simulink model "UberSpurs"  (R2015b)
settings: Solver=VariableStepAuto  StartTime=0.0  StopTime=10000  RelTol=1e-3
(part 4 of 4)

== stateflow chart UberSpurs/spur1WorkCell/route2Channel9/RoutingControlBehavior ==
  (default) -> (junction 7) : % toChanel
  (junction 7) -> (junction 8) [order 1] : [entityChannel == channel && serverAvailable ==0]
  (junction 7) -> (junction 9) [order 2] : {route = 2;}
  (junction 8) -> (junction 10) : {route = 1 ;}
  (junction 10) -> (junction 9)
  (junction 9) -> (junction 11)
  data: entityChannel input; channel input; route output; serverAvailable input

== stateflow chart UberSpurs/spur1WorkCell/route2recirculate/Chart ==
  (default) -> (junction 7) : % recirculate
  (junction 7) -> (junction 9) [order 1] : [FillTime>0]
  (junction 9) -> (junction 23) [order 1] : [verifyQueue<6]
  (junction 9) -> (junction 20) [order 2] : {route = 1;}
  (junction 7) -> (junction 8) [order 2] : {route = 1;}
  (junction 23) -> (junction 25) : {route = 2;}
  (junction 20) -> (junction 8)
  (junction 25) -> (junction 20)
  (junction 8) -> (junction 11)
  data: FillTime input; route output; verifyQueue input

== stateflow chart UberSpurs/AdmissionControlBehavior ==
  (default) -> (junction 7) : % wipLimit
  (junction 7) -> (junction 8) [order 1] : [WIP <= 120]
  (junction 7) -> (junction 9) [order 2] : {admission = 0;}
  (junction 8) -> (junction 10) : {admission = 1;}
  (junction 10) -> (junction 9)
  (junction 9) -> (junction 11)
  data: WIP input; admission output

== stateflow chart UberSpurs/spur1WorkCell/route2Channel10/RoutingControlBehavior ==
  (default) -> (junction 7) : % toChanel
  (junction 7) -> (junction 8) [order 1] : [entityChannel == channel && serverAvailable ==0]
  (junction 7) -> (junction 9) [order 2] : {route = 2;}
  (junction 8) -> (junction 10) : {route = 1 ;}
  (junction 10) -> (junction 9)
  (junction 9) -> (junction 11)
  data: entityChannel input; channel input; route output; serverAvailable input

== stateflow chart UberSpurs/spur1WorkCell/route2Channel11/RoutingControlBehavior ==
  (default) -> (junction 7) : % toChanel
  (junction 7) -> (junction 8) [order 1] : [entityChannel == channel && serverAvailable ==0]
  (junction 7) -> (junction 9) [order 2] : {route = 2;}
  (junction 8) -> (junction 10) : {route = 1 ;}
  (junction 10) -> (junction 9)
  (junction 9) -> (junction 11)
  data: entityChannel input; channel input; route output; serverAvailable input

== stateflow chart UberSpurs/spur1WorkCell/route2Channel12/RoutingControlBehavior ==
  (default) -> (junction 7) : % toChanel
  (junction 7) -> (junction 8) [order 1] : [entityChannel == channel && serverAvailable ==0]
  (junction 7) -> (junction 9) [order 2] : {route = 2;}
  (junction 8) -> (junction 10) : {route = 1 ;}
  (junction 10) -> (junction 9)
  (junction 9) -> (junction 11)
  data: entityChannel input; channel input; route output; serverAvailable input

== stateflow chart UberSpurs/spur1WorkCell/route2Channel13/RoutingControlBehavior ==
  (default) -> (junction 7) : % toChanel
  (junction 7) -> (junction 8) [order 1] : [entityChannel == channel && serverAvailable ==0]
  (junction 7) -> (junction 9) [order 2] : {route = 2;}
  (junction 8) -> (junction 10) : {route = 1 ;}
  (junction 10) -> (junction 9)
  (junction 9) -> (junction 11)
  data: entityChannel input; channel input; route output; serverAvailable input

== stateflow chart UberSpurs/spur1WorkCell/route2Channel14/RoutingControlBehavior ==
  (default) -> (junction 7) : % toChanel
  (junction 7) -> (junction 8) [order 1] : [entityChannel == channel && serverAvailable ==0]
  (junction 7) -> (junction 9) [order 2] : {route = 2;}
  (junction 8) -> (junction 10) : {route = 1 ;}
  (junction 10) -> (junction 9)
  (junction 9) -> (junction 11)
  data: entityChannel input; channel input; route output; serverAvailable input

== stateflow chart UberSpurs/spur1WorkCell/route2Channel15/RoutingControlBehavior ==
  (default) -> (junction 7) : % toChanel
  (junction 7) -> (junction 8) [order 1] : [entityChannel == channel && serverAvailable ==0]
  (junction 7) -> (junction 9) [order 2] : {route = 2;}
  (junction 8) -> (junction 10) : {route = 1 ;}
  (junction 10) -> (junction 9)
  (junction 9) -> (junction 11)
  data: entityChannel input; channel input; route output; serverAvailable input

== stateflow chart UberSpurs/spur1WorkCell/route2Channel16/RoutingControlBehavior ==
  (default) -> (junction 7) : % toChanel
  (junction 7) -> (junction 8) [order 1] : [entityChannel == channel && serverAvailable ==0]
  (junction 7) -> (junction 9) [order 2] : {route = 2;}
  (junction 8) -> (junction 10) : {route = 1 ;}
  (junction 10) -> (junction 9)
  (junction 9) -> (junction 11)
  data: entityChannel input; channel input; route output; serverAvailable input

== stateflow chart UberSpurs/spur1WorkCell/route2Channel17/RoutingControlBehavior ==
  (default) -> (junction 7) : % toChanel
  (junction 7) -> (junction 8) [order 1] : [entityChannel == channel && serverAvailable ==0]
  (junction 7) -> (junction 9) [order 2] : {route = 2;}
  (junction 8) -> (junction 10) : {route = 1 ;}
  (junction 10) -> (junction 9)
  (junction 9) -> (junction 11)
  data: entityChannel input; channel input; route output; serverAvailable input

== stateflow chart UberSpurs/spur1WorkCell/route2Channel18/RoutingControlBehavior ==
  (default) -> (junction 7) : % toChanel
  (junction 7) -> (junction 8) [order 1] : [entityChannel == channel && serverAvailable ==0]
  (junction 7) -> (junction 9) [order 2] : {route = 2;}
  (junction 8) -> (junction 10) : {route = 1 ;}
  (junction 10) -> (junction 9)
  (junction 9) -> (junction 11)
  data: entityChannel input; channel input; route output; serverAvailable input

== stateflow chart UberSpurs/route2Spur2/routingControl ==
  (default) -> (junction 9) : % route2Spur
  (junction 9) -> (junction 10) [order 1] : [entitySpur == 2]
  (junction 9) -> (junction 11) [order 2] : {route = 1;}
  (junction 10) -> (junction 12) : {route = 2;}
  (junction 12) -> (junction 11)
  (junction 11) -> (junction 13)
  data: entitySpur input; route output

== stateflow chart UberSpurs/spur2WorkCell/route2Channel1/RoutingControlBehavior ==
  (default) -> (junction 7) : % toChanel
  (junction 7) -> (junction 8) [order 1] : [entityChannel == channel && serverAvailable ==0]
  (junction 7) -> (junction 9) [order 2] : {route = 2;}
  (junction 8) -> (junction 10) : {route = 1 ;}
  (junction 10) -> (junction 9)
  (junction 9) -> (junction 11)
  data: entityChannel input; channel input; route output; serverAvailable input

== stateflow chart UberSpurs/spur2WorkCell/route2Channel10/RoutingControlBehavior ==
  (default) -> (junction 7) : % toChanel
  (junction 7) -> (junction 8) [order 1] : [entityChannel == channel && serverAvailable ==0]
  (junction 7) -> (junction 9) [order 2] : {route = 2;}
  (junction 8) -> (junction 10) : {route = 1 ;}
  (junction 10) -> (junction 9)
  (junction 9) -> (junction 11)
  data: entityChannel input; channel input; route output; serverAvailable input

== stateflow chart UberSpurs/spur2WorkCell/route2Channel11/RoutingControlBehavior ==
  (default) -> (junction 7) : % toChanel
  (junction 7) -> (junction 8) [order 1] : [entityChannel == channel && serverAvailable ==0]
  (junction 7) -> (junction 9) [order 2] : {route = 2;}
  (junction 8) -> (junction 10) : {route = 1 ;}
  (junction 10) -> (junction 9)
  (junction 9) -> (junction 11)
  data: entityChannel input; channel input; route output; serverAvailable input

== stateflow chart UberSpurs/spur2WorkCell/route2Channel12/RoutingControlBehavior ==
  (default) -> (junction 7) : % toChanel
  (junction 7) -> (junction 8) [order 1] : [entityChannel == channel && serverAvailable ==0]
  (junction 7) -> (junction 9) [order 2] : {route = 2;}
  (junction 8) -> (junction 10) : {route = 1 ;}
  (junction 10) -> (junction 9)
  (junction 9) -> (junction 11)
  data: entityChannel input; channel input; route output; serverAvailable input

== stateflow chart UberSpurs/spur2WorkCell/route2Channel13/RoutingControlBehavior ==
  (default) -> (junction 7) : % toChanel
  (junction 7) -> (junction 8) [order 1] : [entityChannel == channel && serverAvailable ==0]
  (junction 7) -> (junction 9) [order 2] : {route = 2;}
  (junction 8) -> (junction 10) : {route = 1 ;}
  (junction 10) -> (junction 9)
  (junction 9) -> (junction 11)
  data: entityChannel input; channel input; route output; serverAvailable input

== stateflow chart UberSpurs/spur2WorkCell/route2Channel14/RoutingControlBehavior ==
  (default) -> (junction 7) : % toChanel
  (junction 7) -> (junction 8) [order 1] : [entityChannel == channel && serverAvailable ==0]
  (junction 7) -> (junction 9) [order 2] : {route = 2;}
  (junction 8) -> (junction 10) : {route = 1 ;}
  (junction 10) -> (junction 9)
  (junction 9) -> (junction 11)
  data: entityChannel input; channel input; route output; serverAvailable input

== stateflow chart UberSpurs/spur2WorkCell/route2Channel15/RoutingControlBehavior ==
  (default) -> (junction 7) : % toChanel
  (junction 7) -> (junction 8) [order 1] : [entityChannel == channel && serverAvailable ==0]
  (junction 7) -> (junction 9) [order 2] : {route = 2;}
  (junction 8) -> (junction 10) : {route = 1 ;}
  (junction 10) -> (junction 9)
  (junction 9) -> (junction 11)
  data: entityChannel input; channel input; route output; serverAvailable input

== stateflow chart UberSpurs/spur2WorkCell/route2Channel16/RoutingControlBehavior ==
  (default) -> (junction 7) : % toChanel
  (junction 7) -> (junction 8) [order 1] : [entityChannel == channel && serverAvailable ==0]
  (junction 7) -> (junction 9) [order 2] : {route = 2;}
  (junction 8) -> (junction 10) : {route = 1 ;}
  (junction 10) -> (junction 9)
  (junction 9) -> (junction 11)
  data: entityChannel input; channel input; route output; serverAvailable input

== stateflow chart UberSpurs/spur2WorkCell/route2Channel17/RoutingControlBehavior ==
  (default) -> (junction 7) : % toChanel
  (junction 7) -> (junction 8) [order 1] : [entityChannel == channel && serverAvailable ==0]
  (junction 7) -> (junction 9) [order 2] : {route = 2;}
  (junction 8) -> (junction 10) : {route = 1 ;}
  (junction 10) -> (junction 9)
  (junction 9) -> (junction 11)
  data: entityChannel input; channel input; route output; serverAvailable input

== stateflow chart UberSpurs/spur2WorkCell/route2Channel18/RoutingControlBehavior ==
  (default) -> (junction 7) : % toChanel
  (junction 7) -> (junction 8) [order 1] : [entityChannel == channel && serverAvailable ==0]
  (junction 7) -> (junction 9) [order 2] : {route = 2;}
  (junction 8) -> (junction 10) : {route = 1 ;}
  (junction 10) -> (junction 9)
  (junction 9) -> (junction 11)
  data: entityChannel input; channel input; route output; serverAvailable input

== stateflow chart UberSpurs/spur2WorkCell/route2Channel2/RoutingControlBehavior ==
  (default) -> (junction 7) : % toChanel
  (junction 7) -> (junction 8) [order 1] : [entityChannel == channel && serverAvailable ==0]
  (junction 7) -> (junction 9) [order 2] : {route = 2;}
  (junction 8) -> (junction 10) : {route = 1 ;}
  (junction 10) -> (junction 9)
  (junction 9) -> (junction 11)
  data: entityChannel input; channel input; route output; serverAvailable input

== stateflow chart UberSpurs/spur2WorkCell/route2Channel3/RoutingControlBehavior ==
  (default) -> (junction 7) : % toChanel
  (junction 7) -> (junction 8) [order 1] : [entityChannel == channel && serverAvailable ==0]
  (junction 7) -> (junction 9) [order 2] : {route = 2;}
  (junction 8) -> (junction 10) : {route = 1 ;}
  (junction 10) -> (junction 9)
  (junction 9) -> (junction 11)
  data: entityChannel input; channel input; route output; serverAvailable input

== stateflow chart UberSpurs/spur2WorkCell/route2Channel4/RoutingControlBehavior ==
  (default) -> (junction 7) : % toChanel
  (junction 7) -> (junction 8) [order 1] : [entityChannel == channel && serverAvailable ==0]
  (junction 7) -> (junction 9) [order 2] : {route = 2;}
  (junction 8) -> (junction 10) : {route = 1 ;}
  (junction 10) -> (junction 9)
  (junction 9) -> (junction 11)
  data: entityChannel input; channel input; route output; serverAvailable input

== stateflow chart UberSpurs/spur2WorkCell/route2Channel5/RoutingControlBehavior ==
  (default) -> (junction 7) : % toChanel
  (junction 7) -> (junction 8) [order 1] : [entityChannel == channel && serverAvailable ==0]
  (junction 7) -> (junction 9) [order 2] : {route = 2;}
  (junction 8) -> (junction 10) : {route = 1 ;}
  (junction 10) -> (junction 9)
  (junction 9) -> (junction 11)
  data: entityChannel input; channel input; route output; serverAvailable input

== stateflow chart UberSpurs/spur2WorkCell/route2Channel6/RoutingControlBehavior ==
  (default) -> (junction 7) : % toChanel
  (junction 7) -> (junction 8) [order 1] : [entityChannel == channel && serverAvailable ==0]
  (junction 7) -> (junction 9) [order 2] : {route = 2;}
  (junction 8) -> (junction 10) : {route = 1 ;}
  (junction 10) -> (junction 9)
  (junction 9) -> (junction 11)
  data: entityChannel input; channel input; route output; serverAvailable input

== stateflow chart UberSpurs/spur2WorkCell/route2Channel7/RoutingControlBehavior ==
  (default) -> (junction 7) : % toChanel
  (junction 7) -> (junction 8) [order 1] : [entityChannel == channel && serverAvailable ==0]
  (junction 7) -> (junction 9) [order 2] : {route = 2;}
  (junction 8) -> (junction 10) : {route = 1 ;}
  (junction 10) -> (junction 9)
  (junction 9) -> (junction 11)
  data: entityChannel input; channel input; route output; serverAvailable input

== stateflow chart UberSpurs/spur2WorkCell/route2Channel8/RoutingControlBehavior ==
  (default) -> (junction 7) : % toChanel
  (junction 7) -> (junction 8) [order 1] : [entityChannel == channel && serverAvailable ==0]
  (junction 7) -> (junction 9) [order 2] : {route = 2;}
  (junction 8) -> (junction 10) : {route = 1 ;}
  (junction 10) -> (junction 9)
  (junction 9) -> (junction 11)
  data: entityChannel input; channel input; route output; serverAvailable input

== stateflow chart UberSpurs/spur2WorkCell/route2Channel9/RoutingControlBehavior ==
  (default) -> (junction 7) : % toChanel
  (junction 7) -> (junction 8) [order 1] : [entityChannel == channel && serverAvailable ==0]
  (junction 7) -> (junction 9) [order 2] : {route = 2;}
  (junction 8) -> (junction 10) : {route = 1 ;}
  (junction 10) -> (junction 9)
  (junction 9) -> (junction 11)
  data: entityChannel input; channel input; route output; serverAvailable input

== stateflow chart UberSpurs/spur2WorkCell/route2recirculate/Chart ==
  (default) -> (junction 7) : % recirculate
  (junction 7) -> (junction 9) [order 1] : [FillTime>0]
  (junction 9) -> (junction 23) [order 1] : [verifyQueue<6]
  (junction 9) -> (junction 20) [order 2] : {route = 1;}
  (junction 7) -> (junction 8) [order 2] : {route = 1;}
  (junction 23) -> (junction 25) : {route = 2;}
  (junction 20) -> (junction 8)
  (junction 25) -> (junction 20)
  (junction 8) -> (junction 11)
  data: FillTime input; route output; verifyQueue input

== stateflow chart UberSpurs/route2Spur3/routingControl ==
  (default) -> (junction 9) : % route2Spur
  (junction 9) -> (junction 10) [order 1] : [entitySpur == 3]
  (junction 9) -> (junction 11) [order 2] : {route = 1;}
  (junction 10) -> (junction 12) : {route = 2;}
  (junction 12) -> (junction 11)
  (junction 11) -> (junction 13)
  data: entitySpur input; route output

== stateflow chart UberSpurs/spur3WorkCell/route2Channel1/RoutingControlBehavior ==
  (default) -> (junction 7) : % toChanel
  (junction 7) -> (junction 8) [order 1] : [entityChannel == channel && serverAvailable ==0]
  (junction 7) -> (junction 9) [order 2] : {route = 2;}
  (junction 8) -> (junction 10) : {route = 1 ;}
  (junction 10) -> (junction 9)
  (junction 9) -> (junction 11)
  data: entityChannel input; channel input; route output; serverAvailable input

== stateflow chart UberSpurs/spur3WorkCell/route2Channel10/RoutingControlBehavior ==
  (default) -> (junction 7) : % toChanel
  (junction 7) -> (junction 8) [order 1] : [entityChannel == channel && serverAvailable ==0]
  (junction 7) -> (junction 9) [order 2] : {route = 2;}
  (junction 8) -> (junction 10) : {route = 1 ;}
  (junction 10) -> (junction 9)
  (junction 9) -> (junction 11)
  data: entityChannel input; channel input; route output; serverAvailable input

== stateflow chart UberSpurs/spur3WorkCell/route2Channel11/RoutingControlBehavior ==
  (default) -> (junction 7) : % toChanel
  (junction 7) -> (junction 8) [order 1] : [entityChannel == channel && serverAvailable ==0]
  (junction 7) -> (junction 9) [order 2] : {route = 2;}
  (junction 8) -> (junction 10) : {route = 1 ;}
  (junction 10) -> (junction 9)
  (junction 9) -> (junction 11)
  data: entityChannel input; channel input; route output; serverAvailable input

== stateflow chart UberSpurs/spur3WorkCell/route2Channel12/RoutingControlBehavior ==
  (default) -> (junction 7) : % toChanel
  (junction 7) -> (junction 8) [order 1] : [entityChannel == channel && serverAvailable ==0]
  (junction 7) -> (junction 9) [order 2] : {route = 2;}
  (junction 8) -> (junction 10) : {route = 1 ;}
  (junction 10) -> (junction 9)
  (junction 9) -> (junction 11)
  data: entityChannel input; channel input; route output; serverAvailable input

== stateflow chart UberSpurs/spur3WorkCell/route2Channel13/RoutingControlBehavior ==
  (default) -> (junction 7) : % toChanel
  (junction 7) -> (junction 8) [order 1] : [entityChannel == channel && serverAvailable ==0]
  (junction 7) -> (junction 9) [order 2] : {route = 2;}
  (junction 8) -> (junction 10) : {route = 1 ;}
  (junction 10) -> (junction 9)
  (junction 9) -> (junction 11)
  data: entityChannel input; channel input; route output; serverAvailable input

== stateflow chart UberSpurs/spur3WorkCell/route2Channel14/RoutingControlBehavior ==
  (default) -> (junction 7) : % toChanel
  (junction 7) -> (junction 8) [order 1] : [entityChannel == channel && serverAvailable ==0]
  (junction 7) -> (junction 9) [order 2] : {route = 2;}
  (junction 8) -> (junction 10) : {route = 1 ;}
  (junction 10) -> (junction 9)
  (junction 9) -> (junction 11)
  data: entityChannel input; channel input; route output; serverAvailable input

== stateflow chart UberSpurs/spur3WorkCell/route2Channel15/RoutingControlBehavior ==
  (default) -> (junction 7) : % toChanel
  (junction 7) -> (junction 8) [order 1] : [entityChannel == channel && serverAvailable ==0]
  (junction 7) -> (junction 9) [order 2] : {route = 2;}
  (junction 8) -> (junction 10) : {route = 1 ;}
  (junction 10) -> (junction 9)
  (junction 9) -> (junction 11)
  data: entityChannel input; channel input; route output; serverAvailable input

== stateflow chart UberSpurs/spur3WorkCell/route2Channel16/RoutingControlBehavior ==
  (default) -> (junction 7) : % toChanel
  (junction 7) -> (junction 8) [order 1] : [entityChannel == channel && serverAvailable ==0]
  (junction 7) -> (junction 9) [order 2] : {route = 2;}
  (junction 8) -> (junction 10) : {route = 1 ;}
  (junction 10) -> (junction 9)
  (junction 9) -> (junction 11)
  data: entityChannel input; channel input; route output; serverAvailable input

== stateflow chart UberSpurs/spur3WorkCell/route2Channel17/RoutingControlBehavior ==
  (default) -> (junction 7) : % toChanel
  (junction 7) -> (junction 8) [order 1] : [entityChannel == channel && serverAvailable ==0]
  (junction 7) -> (junction 9) [order 2] : {route = 2;}
  (junction 8) -> (junction 10) : {route = 1 ;}
  (junction 10) -> (junction 9)
  (junction 9) -> (junction 11)
  data: entityChannel input; channel input; route output; serverAvailable input

== stateflow chart UberSpurs/spur3WorkCell/route2Channel18/RoutingControlBehavior ==
  (default) -> (junction 7) : % toChanel
  (junction 7) -> (junction 8) [order 1] : [entityChannel == channel && serverAvailable ==0]
  (junction 7) -> (junction 9) [order 2] : {route = 2;}
  (junction 8) -> (junction 10) : {route = 1 ;}
  (junction 10) -> (junction 9)
  (junction 9) -> (junction 11)
  data: entityChannel input; channel input; route output; serverAvailable input

== stateflow chart UberSpurs/spur3WorkCell/route2Channel2/RoutingControlBehavior ==
  (default) -> (junction 7) : % toChanel
  (junction 7) -> (junction 8) [order 1] : [entityChannel == channel && serverAvailable ==0]
  (junction 7) -> (junction 9) [order 2] : {route = 2;}
  (junction 8) -> (junction 10) : {route = 1 ;}
  (junction 10) -> (junction 9)
  (junction 9) -> (junction 11)
  data: entityChannel input; channel input; route output; serverAvailable input

== stateflow chart UberSpurs/spur3WorkCell/route2Channel3/RoutingControlBehavior ==
  (default) -> (junction 7) : % toChanel
  (junction 7) -> (junction 8) [order 1] : [entityChannel == channel && serverAvailable ==0]
  (junction 7) -> (junction 9) [order 2] : {route = 2;}
  (junction 8) -> (junction 10) : {route = 1 ;}
  (junction 10) -> (junction 9)
  (junction 9) -> (junction 11)
  data: entityChannel input; channel input; route output; serverAvailable input

== stateflow chart UberSpurs/spur3WorkCell/route2Channel4/RoutingControlBehavior ==
  (default) -> (junction 7) : % toChanel
  (junction 7) -> (junction 8) [order 1] : [entityChannel == channel && serverAvailable ==0]
  (junction 7) -> (junction 9) [order 2] : {route = 2;}
  (junction 8) -> (junction 10) : {route = 1 ;}
  (junction 10) -> (junction 9)
  (junction 9) -> (junction 11)
  data: entityChannel input; channel input; route output; serverAvailable input

== stateflow chart UberSpurs/spur3WorkCell/route2Channel5/RoutingControlBehavior ==
  (default) -> (junction 7) : % toChanel
  (junction 7) -> (junction 8) [order 1] : [entityChannel == channel && serverAvailable ==0]
  (junction 7) -> (junction 9) [order 2] : {route = 2;}
  (junction 8) -> (junction 10) : {route = 1 ;}
  (junction 10) -> (junction 9)
  (junction 9) -> (junction 11)
  data: entityChannel input; channel input; route output; serverAvailable input

== stateflow chart UberSpurs/spur3WorkCell/route2Channel6/RoutingControlBehavior ==
  (default) -> (junction 7) : % toChanel
  (junction 7) -> (junction 8) [order 1] : [entityChannel == channel && serverAvailable ==0]
  (junction 7) -> (junction 9) [order 2] : {route = 2;}
  (junction 8) -> (junction 10) : {route = 1 ;}
  (junction 10) -> (junction 9)
  (junction 9) -> (junction 11)
  data: entityChannel input; channel input; route output; serverAvailable input

== stateflow chart UberSpurs/spur3WorkCell/route2Channel7/RoutingControlBehavior ==
  (default) -> (junction 7) : % toChanel
  (junction 7) -> (junction 8) [order 1] : [entityChannel == channel && serverAvailable ==0]
  (junction 7) -> (junction 9) [order 2] : {route = 2;}
  (junction 8) -> (junction 10) : {route = 1 ;}
  (junction 10) -> (junction 9)
  (junction 9) -> (junction 11)
  data: entityChannel input; channel input; route output; serverAvailable input

== stateflow chart UberSpurs/spur3WorkCell/route2Channel8/RoutingControlBehavior ==
  (default) -> (junction 7) : % toChanel
  (junction 7) -> (junction 8) [order 1] : [entityChannel == channel && serverAvailable ==0]
  (junction 7) -> (junction 9) [order 2] : {route = 2;}
  (junction 8) -> (junction 10) : {route = 1 ;}
  (junction 10) -> (junction 9)
  (junction 9) -> (junction 11)
  data: entityChannel input; channel input; route output; serverAvailable input

== stateflow chart UberSpurs/spur3WorkCell/route2Channel9/RoutingControlBehavior ==
  (default) -> (junction 7) : % toChanel
  (junction 7) -> (junction 8) [order 1] : [entityChannel == channel && serverAvailable ==0]
  (junction 7) -> (junction 9) [order 2] : {route = 2;}
  (junction 8) -> (junction 10) : {route = 1 ;}
  (junction 10) -> (junction 9)
  (junction 9) -> (junction 11)
  data: entityChannel input; channel input; route output; serverAvailable input

== stateflow chart UberSpurs/spur3WorkCell/route2recirculate/Chart ==
  (default) -> (junction 7) : % recirculate
  (junction 7) -> (junction 9) [order 1] : [FillTime>0]
  (junction 9) -> (junction 23) [order 1] : [verifyQueue<6]
  (junction 9) -> (junction 20) [order 2] : {route = 1;}
  (junction 7) -> (junction 8) [order 2] : {route = 1;}
  (junction 23) -> (junction 25) : {route = 2;}
  (junction 20) -> (junction 8)
  (junction 25) -> (junction 20)
  (junction 8) -> (junction 11)
  data: FillTime input; route output; verifyQueue input
